simulink model "FiltroDigital"  (R2023b)
settings: Solver=VariableStepAuto  StartTime=0.0  StopTime=0.3  RelTol=1e-3
undefined symbols (not defined in the file): analogCircuit
libraries: slctrl_linear x1, dspmlti4 x1
settings Model: Creator=elias  LastModifiedBy=elias

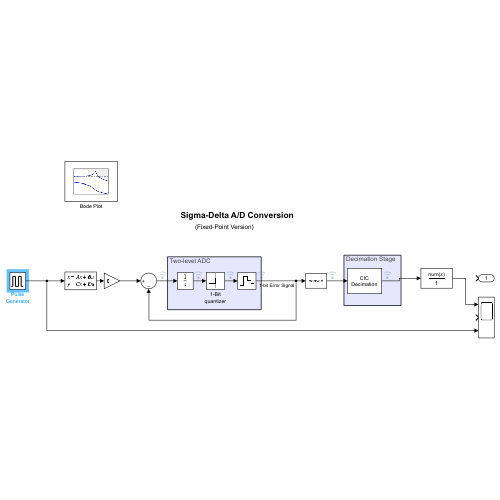
[thumbnail: Simulink's stored preview of the top-level diagram]
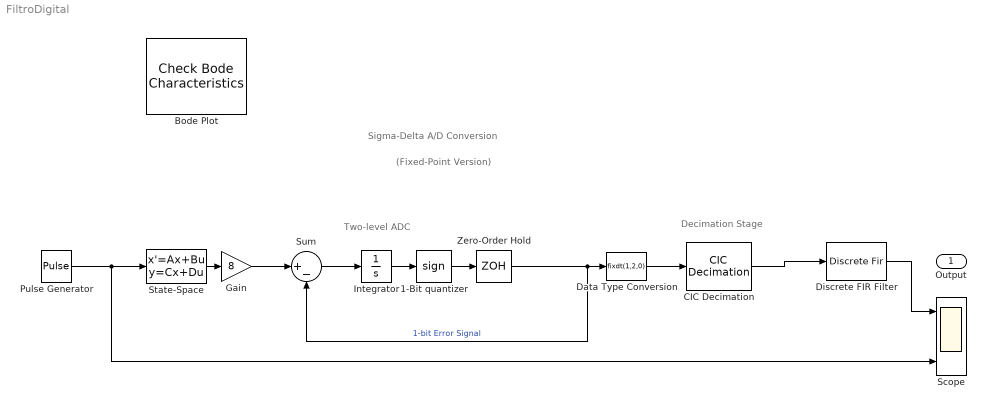
== system FiltroDigital ==
  note: (Fixed-Point Version)
  note: Two-level ADC
  note: Decimation Stage
  note: Sigma-Delta A/D Conversion
  1-Bit quantizer : Signum
  Bode Plot : slctrl_linear/Check Bode  Characteristics  InstantiateOnLoad=on  SaveOperatingPoints=off  LinearizationIOs={'/Pulse Generator', 1, 'in', 'off', '';'/Discrete FIR Filter', 1, 'out', 'off', ''}  LinearizeAt=SnapshotTimes  SnapshotTimes=[0]  TriggerType=rising  SampleTime=auto  RateConversionMethod=zoh  PreWarpFreq=10  UseExactDelayModel=off  UseFullBlockNameLabels=off  UseBusSignalLabels=off  enabled=on  stopWhenAssertionFail=off  export=off  ViewDlgPos=[922.6 185 509.6 389.6]  OpenViewOnLoad=on  LaunchViewOnOpen=off  FrequencyUnits=rad/s  MagnitudeUnits=dB  PhaseUnits=deg  TimeUnits=seconds  EnableUpperBound=off  UpperBoundFrequencies=[]  UpperBoundMagnitudes=[]  EnableLowerBound=off  LowerBoundFrequencies=[]  LowerBoundMagnitudes=[]
      settings: LibrarySourceBlock=slctrlblks/Linear Analysis Plots/Bode Plot  SaveToWorkspace=off  SaveName=sys
  CIC Decimation : dspmlti4/CIC Decimation  filtFrom=Dialog parameters  filtobj=Hm_decim  ftype=Decimator  R=64  M=1  N=5  filterInternals=Full precision  BPS=[32 30 24 20 16 16 16 16 16 16]  FLPS=0  outputWordLength=16  outputFracLength=0  launchFVT=off  framing=Maintain input frame rate  RateOptions=Allow multirate processing
  Data Type Conversion : DataTypeConversion  OutDataTypeStr=fixdt(1,2,0)  SaturateOnIntegerOverflow=off  RndMeth=Floor
  Discrete FIR Filter : DiscreteFir  Coefficients=fir1(127, [(240 - 27/2), (240 + 27/2)] / (1488 / 2))
  Gain : Gain  Gain=8
  Integrator : Integrator
  Pulse Generator : DiscretePulseGenerator  PulseType=Time based  Period=0.5  PulseWidth=50
  Scope : Scope  NumInputPorts=3
  State-Space : StateSpace  A=analogCircuit.A  B=analogCircuit.B  C=analogCircuit.C  D=analogCircuit.D  InitialCondition=0
  Sum : Sum  Inputs=|+-  InputSameDT=on  SaturateOnIntegerOverflow=on  OutDataTypeStr=Inherit: Same as first input
  Zero-Order Hold : ZeroOrderHold  SampleTime=1/384e3
  Output : Outport
  wires:
  CIC Decimation/1 -> Discrete FIR Filter/1
  Sum/1 -> Integrator/1
  Data Type Conversion/1 -> CIC Decimation/1
  Integrator/1 -> 1-Bit quantizer/1
  Zero-Order Hold/1 -> Data Type Conversion/1, Sum/2  "1-bit Error Signal"
  1-Bit quantizer/1 -> Zero-Order Hold/1
  Pulse Generator/1 -> Scope/3, State-Space/1
  State-Space/1 -> Gain/1
  Gain/1 -> Sum/1
  Discrete FIR Filter/1 -> Scope/1
